simulink model "test_lsq_sim3_ok"  (R2020b)
settings: Solver=VariableStepAuto  StartTime=0.0  StopTime=1  RelTol=1e-3  EnableMultiTasking=on
values from neighbouring files (symbols this model uses):
  b = 5    [elip_test.m]    (also in ellip_force_test.m = 4; multi_sim2.m = FM(:,i))
  c_mat = [alligned_Force_vectors;Moment_Vectors']    [control_mat.m]
  N_sat = length(azimuths)    [ellip_force_test.m]    (also in initial_sim.m = 30; initial_sim2.m = 25; multi_sim.m = sim_data.N_sat; multi_sim2.m = sim_data.N_sat)
settings Model: RequirementInfo="{}  %GIDa_6cedf146_90b2_42a8_8a44_863cb2ad063c"  Creator=hamzaali  LastModifiedBy=Mehdi
settings DataIOCC: ReturnWorkspaceOutputs=off
settings OptimizationCC: LifeSpan=inf
settings DebuggingCC: SFUnexpectedBacktrackingDiag=warning  SFNoUnconditionalDefaultTransitionDiag=warning  ArithmeticOperatorsInVariantConditions=warning
settings SFSimCC: SimUseLocalCustomCode=off  CustomCodeUndefinedFunction=UseInterfaceOnly
settings RTWCC: RTWUseLocalCustomCode=off
settings CodeAppCC: StateflowObjectComments=on
settings GRTTargetCC: TargetLangStandard=C89/C90 (ANSI)
settings ConfigComp: CovMetricSettings=dw  CovSaveCumulativeToWorkspaceVar=on  CovSaveSingleToWorkspaceVar=on  CovExternalEMLEnable=off

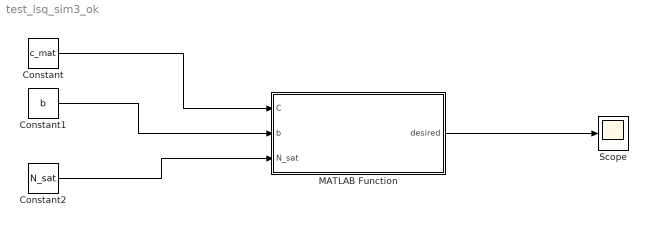
== system test_lsq_sim3_ok ==
  Constant : Constant  Value=c_mat
  Constant1 : Constant  Value=b
  Constant2 : Constant  Value=N_sat
  MATLAB Function : MATLAB Function  TreatAsAtomicUnit=on
  Scope : Scope
  wires:
  MATLAB Function/1(desired) -> Scope/1
  Constant1/1 -> MATLAB Function/2(b)
  Constant2/1 -> MATLAB Function/3(N_sat)
  Constant/1 -> MATLAB Function/1(C)

== matlab function test_lsq_sim3_ok/MATLAB Function ==
  settings: updateMethod=DISCRETE  sampleTime=0.001
  data: C input; desired output size=[40]; b input; N_sat input
function desired = path_planning(C,b,N_sat)



desired=zeros(N_sat,1);


f=ones(1,N_sat);
lb=zeros(N_sat,1);
ub=ones(N_sat,1)*inf;
% % options = optimset('TolX',1e-20);
% options = optimset;
% options.MaxIter=200;
% options.Display='none';

[desired,exitflag] = new_linprog(f,C,b,lb,ub);

% for i=1:N_sat
%     out1(i)=x(i);
% end




end
